simulink model "MIMO_RSLQR_2020"  (R2022a)
settings: Solver=VariableStepAuto  StartTime=0.0  StopTime=50  RelTol=1e-3
values from neighbouring files (symbols this model uses):
  Ap = Ap( 1:2, 1:2)    [Adaptive_OBLTR_hmk9_2020.m]    (also in Bicycle_Model_Controller.m = [0 1 0 0; H2_P1.m = [ -0.576007 -3255.07 4.88557 9.25796; H2_P3.m = [ZaV 1; Ma 0]; H3_P1.m = [Za_V  1.      Zd_V          0.)
  Bp = Bp( 1:2)    [Adaptive_OBLTR_hmk9_2020.m]    (also in Bicycle_Model_Controller.m = [B_d B_psi]; H2_P1.m = [ 0 ; 0 ; 0 ; 8882.64]; H2_P3.m = [ZdV; Md]; H3_P1.m = [0.; 0.; 0.; w_act*w_act ])
  C = [1 0 0 0 0 ... (first row only)    [Hmk5_output_feedback.m]    (also in Hmk6_OBLTR.m = [1 0 0; 0 0 1]; MIMO_RSLQR_Test.m = [1 0 0 0; 0 1 0 0]; square_system_inputs_pp.m = sys_orig.c)
  Cp = eye(2)    [Adaptive_OBLTR_hmk9_2020.m]    (also in Bicycle_Model_Controller.m = eye(nx); H2_P1.m = [ 1 0 0 0; H2_P3.m = [Za 0; 0 1]; H3_P1.m = [  Za   0.  Zd  0.)
  K_I = Kx_lqr(:,1:2)    [MIMO_RSLQR_Test.m]
  K_X = Kx_lqr(:,3:6)    [MIMO_RSLQR_Test.m]
settings Model: Creator=F87909D  LastModifiedBy=F87909D
settings SolverCC: AlgebraicLoopSolver=TrustRegion
settings DebuggingCC: UnconnectedInputMsg=warning  UnconnectedOutputMsg=warning  UnconnectedLineMsg=warning  SFMachineParentedDataDiag=warning
settings RTWCC: DLArmComputeVersion=19.05

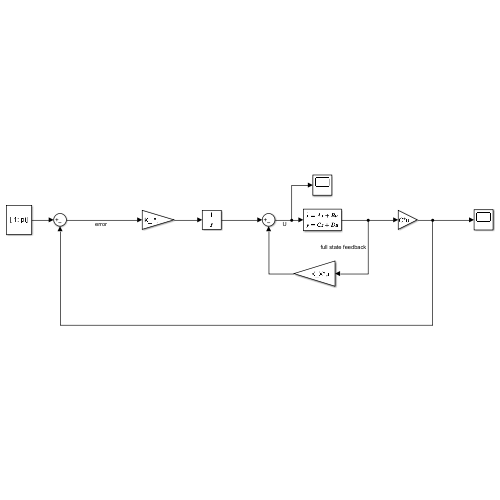
[thumbnail: Simulink's stored preview of the top-level diagram]
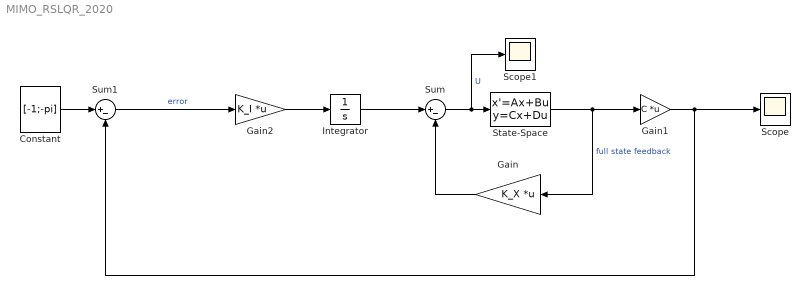
== system MIMO_RSLQR_2020 ==
  Constant : Constant  Value=[-1;-pi]
  Gain : Gain  Gain=K_X  Multiplication=Matrix(K*u)
  Gain1 : Gain  Gain=C  Multiplication=Matrix(K*u)
  Gain2 : Gain  Gain=K_I  Multiplication=Matrix(K*u)
  Integrator : Integrator
  Scope : Scope
  Scope1 : Scope
  State-Space : StateSpace  A=Ap  B=Bp  C=Cp  D=0.*Cp*Bp;  InitialCondition=[1; -1; 3.14; 0]
  Sum : Sum  Inputs=|+-
  Sum1 : Sum  Inputs=|+-
  wires:
  State-Space/1 -> Gain1/1, Gain/1  "full state feedback"
  Sum/1 -> Scope1/1, State-Space/1  "U"
  Gain/1 -> Sum/2
  Integrator/1 -> Sum/1
  Gain2/1 -> Integrator/1
  Constant/1 -> Sum1/1
  Sum1/1 -> Gain2/1  "error"
  Gain1/1 -> Scope/1, Sum1/2
